simulink library "uavsimblockset_SixDOFKinematics"  (Simulink 8.4)
settings: Solver=ode45  StartTime=0.0  StopTime=10.0  RelTol=1e-3
undefined symbols (not defined in the file): Earth, fflib_rrm2degdegm, mask_cularis_originNED_ECEF_rrm, mask_cularis_p0_ECEF_lla, mask_cularis_phithetapsi0, mask_cularis_pqr0, mask_cularis_uvw0, uavsim, WGS84
libraries: aerolibobsolete x1, aerolibtransform2 x1, uavsimblockset_vbody2vNED x1
settings Model: Creator=mstolle  LastModifiedBy=j.bolting

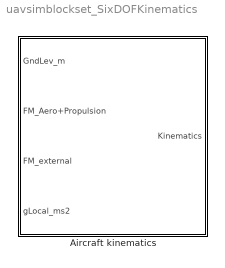
== system uavsimblockset_SixDOFKinematics ==
  Aircraft kinematics : Subsystem  mask{mask_inertia=uavsim.CULARIS.inertiaTensor, mask_mass=uavsim.CULARIS.mass, mask_P0_ECEF_rrm=mask_cularis_p0_ECEF_lla, mask_originNED_ECEF_rrm=mask_cularis_originNED_ECEF_rrm, mask_uvw0=mask_cularis_uvw0, mask_phithetapsi0=mask_cularis_phithetapsi0, mask_omega0=mask_cularis_pqr0}
      mask prompts: mask_inertia "Inertia tensor [kg * m²]"; mask_mass "Aircraft mass [kg]"; mask_P0_ECEF_rrm "Initial ECEF position [rad,rad,m]"; mask_originNED_ECEF_rrm "Origin NED frame, ECEF WGS84, [rad rad m]"; mask_uvw0 "Initial velocity vector, body frame [m/s]"; mask_phithetapsi0 "Initial Euler angles [rad]"; mask_omega0 "Initial body rotation rates [rad/s]"

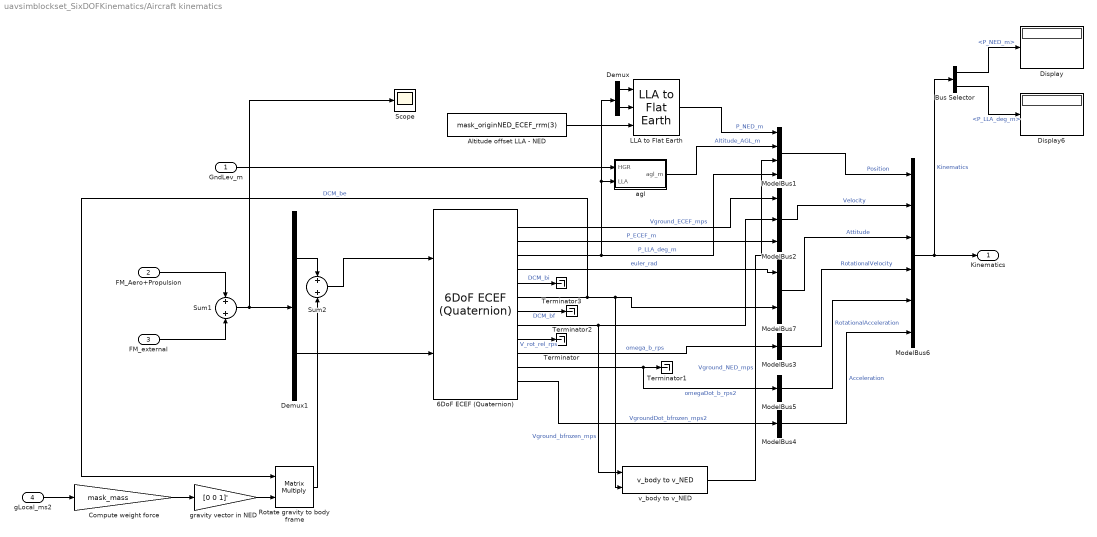
== system uavsimblockset_SixDOFKinematics/Aircraft kinematics ==
  GndLev_m : Inport
  FM_Aero+Propulsion : Inport  Port=2
  FM_external : Inport  Port=3
  gLocal_ms2 : Inport  Port=4
  6DoF ECEF (Quaternion) : aerolibobsolete/6DoF ECEF (Quaternion)  units=Metric (MKS)  mtype=Fixed  xg_0=fflib_rrm2degdegm(mask_P0_ECEF_rrm)  Vm_0=mask_uvw0  eul_0=mask_phithetapsi0  pm_0=mask_omega0  mass_0=mask_mass  mass_e=0.5  mass_f=2.0  inertia=mask_inertia  inertia_e=eye(3)  inertia_f=2*eye(3)  ptype=Earth (WGS84)  F=1/298.257223563  R=6378137  w_E=7292115e-11  angle_in=Internal  LG0=0
  Altitude offset LLA - NED : Constant  Value=mask_originNED_ECEF_rrm(3)
  Bus Selector : BusSelector  OutputSignals=Position.P_NED_m,Position.P_LLA_deg_m
  Compute weight force : Gain  Gain=mask_mass
  Demux : Demux  Outputs=[2 1]
  Demux1 : Demux  Outputs=[3,3]
  Display : Display
  Display6 : Display
  LLA to Flat Earth : aerolibtransform2/LLA to Flat Earth  units=Metric (MKS)  ptype=Earth (WGS84)  F=1/298.257223563  R=6378137  LL0=rad2deg(mask_originNED_ECEF_rrm(1:2))  psi=0
  ModelBus1 : BusCreator  OutDataTypeStr=Bus: Position
  ModelBus2 : BusCreator  Inputs=3  OutDataTypeStr=Bus: Velocity
  ModelBus3 : BusCreator  Inputs=1  OutDataTypeStr=Bus: RotationalVelocity
  ModelBus4 : BusCreator  Inputs=1  OutDataTypeStr=Bus: Acceleration
  ModelBus5 : BusCreator  Inputs=1  OutDataTypeStr=Bus: RotationalAcceleration
  ModelBus6 : BusCreator  Inputs=6  OutDataTypeStr=Bus: Kinematics  NonVirtualBus=on
  ModelBus7 : BusCreator  Inputs=2  OutDataTypeStr=Bus: Attitude
  Rotate gravity to body frame : Product  Multiplication=Matrix(*)
  Scope : Scope
  Sum1 : Sum  SaturateOnIntegerOverflow=on  InputSameDT=on  OutDataTypeStr=Inherit: Same as first input
  Sum2 : Sum  SaturateOnIntegerOverflow=on  InputSameDT=on  OutDataTypeStr=Inherit: Same as first input
  Terminator{,1..3} (4 alike) : Terminator
  agl : Subsystem
  gravity vector in NED : Gain  Gain=[0 0 1]'
  v_body to v_NED : uavsimblockset_vbody2vNED/v_body to v_NED
  Kinematics : Outport  OutDataTypeStr=Bus: Kinematics
  wires:
  6DoF ECEF (Quaternion)/3 -> ModelBus1/4, Demux/1, agl/2(LLA)  "P_LLA_deg_m"
  Bus Selector/2 -> Display6/1  "<P_LLA_deg_m>"
  Bus Selector/1 -> Display/1  "<P_NED_m>"
  6DoF ECEF (Quaternion)/12 -> ModelBus4/1  "VgroundDot_bfrozen_mps2"
  6DoF ECEF (Quaternion)/11 -> Terminator1/1, ModelBus5/1  "omegaDot_b_rps2"
  ModelBus6/1 -> Kinematics/1, Bus Selector/1  "Kinematics"
  6DoF ECEF (Quaternion)/5 -> Terminator3/1  "DCM_bi"
  ModelBus2/1 -> ModelBus6/2  "Velocity"
  ModelBus3/1 -> ModelBus6/4  "RotationalVelocity"
  6DoF ECEF (Quaternion)/2 -> ModelBus1/3  "P_ECEF_m"
  ModelBus5/1 -> ModelBus6/5  "RotationalAcceleration"
  6DoF ECEF (Quaternion)/6 -> Rotate gravity to body frame/1, ModelBus7/2, v_body to v_NED/2  "DCM_be"
  6DoF ECEF (Quaternion)/9 -> Terminator/1  "V_rot_rel_rps"
  6DoF ECEF (Quaternion)/10 -> ModelBus3/1  "omega_b_rps"
  ModelBus7/1 -> ModelBus6/3  "Attitude"
  agl/1(agl_m) -> ModelBus1/2  "Altitude_AGL_m"
  6DoF ECEF (Quaternion)/4 -> ModelBus7/1  "euler_rad"
  LLA to Flat Earth/1 -> ModelBus1/1  "P_NED_m"
  ModelBus1/1 -> ModelBus6/1  "Position"
  6DoF ECEF (Quaternion)/1 -> ModelBus2/1  "Vground_ECEF_mps"
  ModelBus4/1 -> ModelBus6/6  "Acceleration"
  6DoF ECEF (Quaternion)/7 -> Terminator2/1  "DCM_bf"
  6DoF ECEF (Quaternion)/8 -> v_body to v_NED/1, ModelBus2/2  "Vground_bfrozen_mps"
  Demux1/2 -> 6DoF ECEF (Quaternion)/2
  Sum2/1 -> 6DoF ECEF (Quaternion)/1
  Sum1/1 -> Demux1/1, Scope/1
  Demux1/1 -> Sum2/1
  GndLev_m/1 -> agl/1(HGR)
  FM_Aero+Propulsion/1 -> Sum1/1
  FM_external/1 -> Sum1/2
  Demux/1 -> LLA to Flat Earth/1
  Demux/2 -> LLA to Flat Earth/2
  Altitude offset LLA - NED/1 -> LLA to Flat Earth/3
  v_body to v_NED/1 -> ModelBus2/3  "Vground_NED_mps"
  gLocal_ms2/1 -> Compute weight force/1
  gravity vector in NED/1 -> Rotate gravity to body frame/2
  Rotate gravity to body frame/1 -> Sum2/2
  Compute weight force/1 -> gravity vector in NED/1

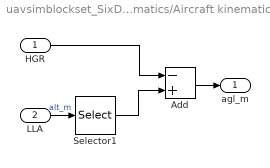
== system uavsimblockset_SixDOFKinematics/Aircraft kinematics/agl ==
  HGR : Inport
  LLA : Inport  Port=2
  Add : Sum  Inputs=-+
  Selector1 : Selector  InputPortWidth=3  Indices=[3]
  agl_m : Outport
  wires:
  HGR/1 -> Add/1
  LLA/1 -> Selector1/1  "alt_m"
  Selector1/1 -> Add/2
  Add/1 -> agl_m/1
